simulink model "stateflow_swing_up_controller"  (R2020b)
settings: Solver=VariableStepAuto  StartTime=0.0  StopTime=30  RelTol=1e-3
libraries: vrlib x1, pid_lib x1
settings Model: Creator=angelo  LastModifiedBy=angel

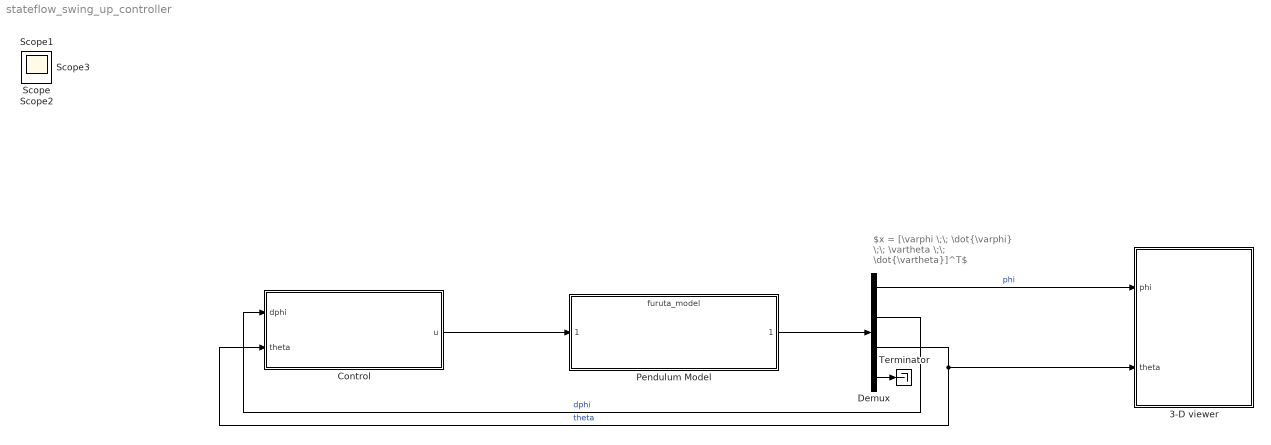
== system stateflow_swing_up_controller ==
  note: $x = [\varphi \;\; \dot{\varphi} \;\; \vartheta \;\; \dot{\vartheta}]^T$
  3-D viewer : Subsystem
  Control : Subsystem
  Demux : Demux
  Pendulum Model : ModelReference  ModelNameDialog=furuta_model.slx  SimulationMode=Normal  ModelReferenceVersion=1.21
  Terminator : Terminator
  Scope{,1..3} (4 alike) : Scope
  wires:
  Pendulum Model/1 -> Demux/1
  Demux/3 -> Control/2(theta), 3-D viewer/2(theta)  "theta"
  Demux/1 -> 3-D viewer/1(phi)  "phi"
  Demux/2 -> Control/1(dphi)  "dphi"
  Control/1(u) -> Pendulum Model/1
  Demux/4 -> Terminator/1

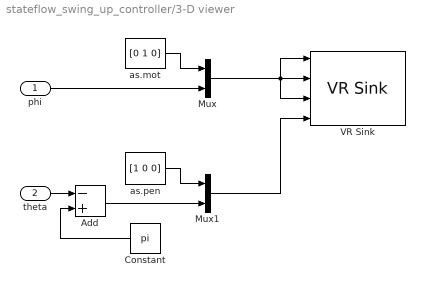
== system stateflow_swing_up_controller/3-D viewer ==
  phi : Inport
  theta : Inport  Port=2
  Add : Sum  Inputs=-+
  Constant : Constant  Value=pi
  Mux : Mux  Inputs=2
  Mux1 : Mux  Inputs=2
  VR Sink : vrlib/VR Sink  InstantiateOnLoad=on  SampleTime=0.02  ViewEnable=on  RemoteChange=off  RemoteView=on  FieldsWritten=Puleggia_8.rotation.4.1.1.double#Puleggia.rotation.4.1.1.double#LinkP-L.rotation.4.1.1.double#pispolo.rotation.4.1.1.double  WorldFileName=fu.wrl  AutoView=off  VideoDimensions=[]  AllowVariableSize=off
  as.mot : Constant  Value=[0 1 0]
  as.pen : Constant  Value=[1 0 0]
  wires:
  as.mot/1 -> Mux/1
  as.pen/1 -> Mux1/1
  Mux/1 -> VR Sink/1, VR Sink/3, VR Sink/2
  Mux1/1 -> VR Sink/4
  Add/1 -> Mux1/2
  Constant/1 -> Add/2
  phi/1 -> Mux/2
  theta/1 -> Add/1

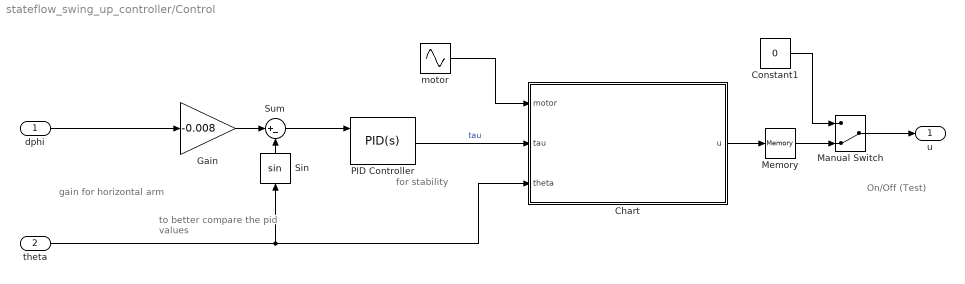
== system stateflow_swing_up_controller/Control ==
  note: to better compare the pid values
  note: On/Off
      | (Test)
  note: for stability
  note: gain for horizontal arm
  dphi : Inport
  theta : Inport  Port=2
  Chart : Stateflow chart  TreatAsAtomicUnit=on  SystemSampleTime=0.01
  Constant1 : Constant  Value=0
  Gain : Gain  Gain=-0.008
  Manual Switch : ManualSwitch  CurrentSetting=0
  Memory : Memory
  PID Controller : pid_lib/PID Controller  Controller=PID  Form=Parallel  TimeDomain=Continuous-time  UseExternalTs=off  SampleTime=-1  IntegratorMethod=Forward Euler  FilterMethod=Forward Euler  ControllerParametersSource=internal  P=-18  I=-25  D=-2.5  UseFilter=on  N=100  TunerSelectOption=Transfer Function Based (PID Tuner App)  InitialConditionSource=internal  InitialConditionForIntegrator=0  InitialConditionForFilter=0  DifferentiatorICPrevScaledInput=0  ExternalReset=level  TrackingMode=off  Kt=1  LimitOutput=on  SatLimitsSource=internal  UpperSaturationLimit=10  LowerSaturationLimit=-10  LinearizeAsGain=on  AntiWindupMode=none  Kb=1  POutMin=[]  POutMax=[]  IOutMin=[]  IOutMax=[]  DOutMin=[]  DOutMax=[]  NOutMin=[]  NOutMax=[]  SumOutMin=[]  SumOutMax=[]  SaturationOutMin=[]  SaturationOutMax=[]  PParamMin=[]  PParamMax=[]  IParamMin=[]  IParamMax=[]  DParamMin=[]  DParamMax=[]  NParamMin=[]  NParamMax=[]  KbParamMin=[]  KbParamMax=[]  KtParamMin=[]  KtParamMax=[]  KbOutMin=[]  KbOutMax=[]  KtOutMin=[]  KtOutMax=[]  IntegratorOutMin=[]  IntegratorOutMax=[]  FilterOutMin=[]  FilterOutMax=[]  SumI1OutMin=[]  SumI1OutMax=[]  SumI2OutMin=[]  SumI2OutMax=[]  SumI3OutMin=[]  SumI3OutMax=[]  SumI4OutMin=[]  SumI4OutMax=[]  SumDOutMin=[]  SumDOutMax=[]  DifferentiatorOutMin=[]  DifferentiatorOutMax=[]  FilterDiffOutCoefMin=[]  FilterDiffOutCoefMax=[]  ReciprocalOutMin=[]  ReciprocalOutMax=[]  SumDenOutMin=[]  SumDenOutMax=[]  SumNumOutMin=[]  SumNumOutMax=[]  DivideOutMin=[]  DivideOutMax=[]  UdiffTsProdOutMin=[]  UdiffTsProdOutMax=[]  NTsProdOutMin=[]  NTsProdOutMax=[]  UintegralTsProdOutMin=[]  UintegralTsProdOutMax=[]  UngainTsProdOutMin=[]  UngainTsProdOutMax=[]  IntegratorContinuousStateAttributes=''  IntegratorStateMustResolveToSignalObject=off  IntegratorRTWStateStorageClass=Auto  FilterContinuousStateAttributes=''  FilterStateMustResolveToSignalObject=off  FilterRTWStateStorageClass=Auto  ParallelPVariant=InternalParameters  IdealPVariant=Disabled  IVariant=InternalParameters  DVariant=InternalParameters  IntegratorVariant=Continuous  SatVariant=Enabled  AWVariant=Passthrough  PCopyVariant=Disabled  TRVariant=Disabled  FdbkBlocksVariant=Forward  IdealPFdbkVariant=Disabled  SatFdbkVariant=Disabled  DerivativeFilterVariant=ContFilter  NVariant=InternalParameters  NCopyVariant=Disabled  FilterICVariant=InternalICsFilter  IntegratorICVariant=InternalICs  ExternalResetVariant=ExternalReset  TRSumVariant=Passthrough  SumFdbkVariant=Disabled  SumVariant=Sum_PID  TsampFilterVariant=InternalTs  TsampNgainVariant=Passthrough  TsampIntegralVariant=Passthrough  ExternalSaturationOutDataTypeStr=Inherit: Same as second input
  Sin : Trigonometry
  Sum : Sum  Inputs=|+-
  motor : Sin  Amplitude=8  Frequency=2*pi  SampleTime=0
  u : Outport
  wires:
  dphi/1 -> Gain/1
  Gain/1 -> Sum/1
  Sum/1 -> PID Controller/1
  Sin/1 -> Sum/2
  Manual Switch/1 -> u/1
  Constant1/1 -> Manual Switch/1
  theta/1 -> Chart/3(theta), Sin/1
  motor/1 -> Chart/1(motor)
  PID Controller/1 -> Chart/2(tau)  "tau"
  Chart/1(u) -> Memory/1
  Memory/1 -> Manual Switch/2

== stateflow chart stateflow_swing_up_controller/Control/Chart ==
  state farZero
    du: u = motor;
  state closeZero
    du: u = tau;
  (default) -> farZero
  farZero -> closeZero : [cos(theta) > cos(pi/8)]
  closeZero -> farZero : [cos(theta) < cos(pi/8)]
  data: motor input; tau input; u output =0; theta input
